simulink model "TST_InjCrv_MI1Cor"  (R2016b)
settings: Solver=FixedStepDiscrete  StartTime=0.0  StopTime=simTime  FixedStep=sampleTime  RelTol=1e-3
values from neighbouring files (symbols this model uses):
  testCase = 1    [initTST_InjCrv_MI1Cor_001.m]
libraries: simulink x3, UnitTest_Lib x1
settings Model: Creator=zhengjinyan  LastModifiedBy=zhengjinyan
settings DebuggingCC: SignalRangeChecking=error

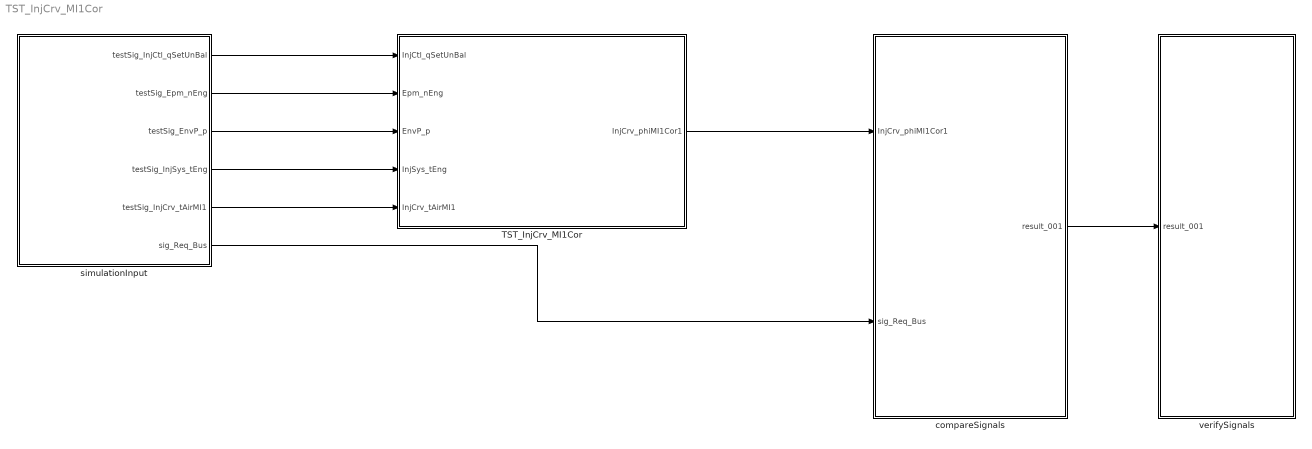
== system TST_InjCrv_MI1Cor ==
  TST_InjCrv_MI1Cor : Subsystem
  compareSignals : Subsystem
  simulationInput : Subsystem
  verifySignals : Subsystem
  wires:
  simulationInput/1(testSig_InjCtl_qSetUnBal) -> TST_InjCrv_MI1Cor/1(InjCtl_qSetUnBal)
  simulationInput/2(testSig_Epm_nEng) -> TST_InjCrv_MI1Cor/2(Epm_nEng)
  simulationInput/3(testSig_EnvP_p) -> TST_InjCrv_MI1Cor/3(EnvP_p)
  simulationInput/4(testSig_InjSys_tEng) -> TST_InjCrv_MI1Cor/4(InjSys_tEng)
  simulationInput/5(testSig_InjCrv_tAirMI1) -> TST_InjCrv_MI1Cor/5(InjCrv_tAirMI1)
  TST_InjCrv_MI1Cor/1(InjCrv_phiMI1Cor1) -> compareSignals/1(InjCrv_phiMI1Cor1)
  simulationInput/6(sig_Req_Bus) -> compareSignals/2(sig_Req_Bus)
  compareSignals/1(result_001) -> verifySignals/1(result_001)

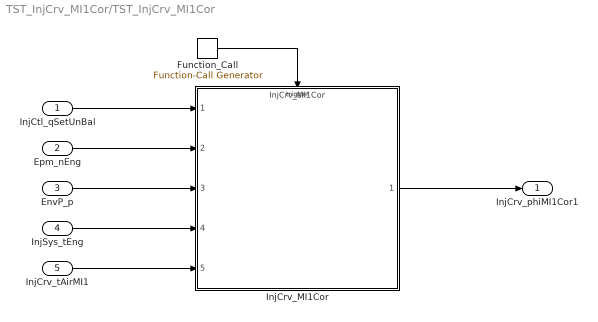
== system TST_InjCrv_MI1Cor/TST_InjCrv_MI1Cor ==
  InjCtl_qSetUnBal : Inport
  Epm_nEng : Inport  Port=2
  EnvP_p : Inport  Port=3
  InjSys_tEng : Inport  Port=4
  InjCrv_tAirMI1 : Inport  Port=5
  Function_Call : simulink/Ports & Subsystems/Function-Call Generator  sample_time=sampleTime  numberOfIterations=1
  InjCrv_MI1Cor : ModelReference  ModelNameDialog=InjCrv_MI1Cor  SimulationMode=Normal  ModelReferenceVersion=1.23  TriggerPortName=function  TriggerPortTriggerType=function-call  TriggerPortStatesWhenEnabling=held
  InjCrv_phiMI1Cor1 : Outport
  wires:
  Function_Call/1 -> InjCrv_MI1Cor/Trigger
  InjCtl_qSetUnBal/1 -> InjCrv_MI1Cor/1
  Epm_nEng/1 -> InjCrv_MI1Cor/2
  EnvP_p/1 -> InjCrv_MI1Cor/3
  InjSys_tEng/1 -> InjCrv_MI1Cor/4
  InjCrv_tAirMI1/1 -> InjCrv_MI1Cor/5
  InjCrv_MI1Cor/1 -> InjCrv_phiMI1Cor1/1

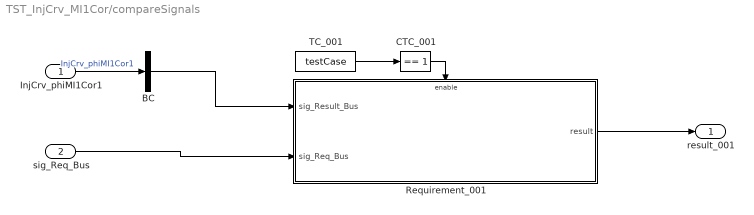
== system TST_InjCrv_MI1Cor/compareSignals ==
  InjCrv_phiMI1Cor1 : Inport
  sig_Req_Bus : Inport  Port=2
  BC : BusCreator  Inputs=1
  CTC_001 : simulink/Logic and Bit Operations/Compare To Constant  relop===  const=1  OutDataTypeStr=boolean
  Requirement_001 : Subsystem
  TC_001 : Constant  Value=testCase
  result_001 : Outport
  wires:
  InjCrv_phiMI1Cor1/1 -> BC/1  "InjCrv_phiMI1Cor1"
  TC_001/1 -> CTC_001/1
  CTC_001/1 -> Requirement_001/Enable
  sig_Req_Bus/1 -> Requirement_001/2(sig_Req_Bus)
  BC/1 -> Requirement_001/1(sig_Result_Bus)
  Requirement_001/1(result) -> result_001/1

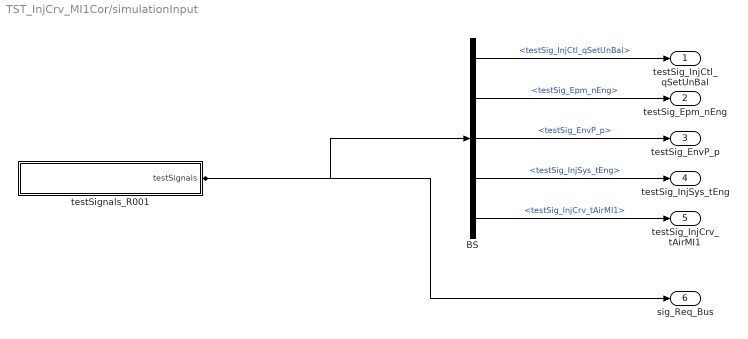
== system TST_InjCrv_MI1Cor/simulationInput ==
  BS : BusSelector  OutputSignals=testSig_InjCtl_qSetUnBal,testSig_Epm_nEng,testSig_EnvP_p,testSig_InjSys_tEng,testSig_InjCrv_tAirMI1
  testSignals_R001 : Subsystem
  testSig_InjCtl_qSetUnBal : Outport
  testSig_Epm_nEng : Outport  Port=2
  testSig_EnvP_p : Outport  Port=3
  testSig_InjSys_tEng : Outport  Port=4
  testSig_InjCrv_tAirMI1 : Outport  Port=5
  sig_Req_Bus : Outport  Port=6
  wires:
  BS/1 -> testSig_InjCtl_qSetUnBal/1  "<testSig_InjCtl_qSetUnBal>"
  BS/2 -> testSig_Epm_nEng/1  "<testSig_Epm_nEng>"
  BS/3 -> testSig_EnvP_p/1  "<testSig_EnvP_p>"
  BS/4 -> testSig_InjSys_tEng/1  "<testSig_InjSys_tEng>"
  BS/5 -> testSig_InjCrv_tAirMI1/1  "<testSig_InjCrv_tAirMI1>"
  testSignals_R001/1(testSignals) -> BS/1, sig_Req_Bus/1

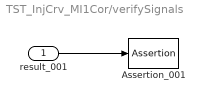
== system TST_InjCrv_MI1Cor/verifySignals ==
  result_001 : Inport
  Assertion_001 : Assertion  Enabled=off
  wires:
  result_001/1 -> Assertion_001/1

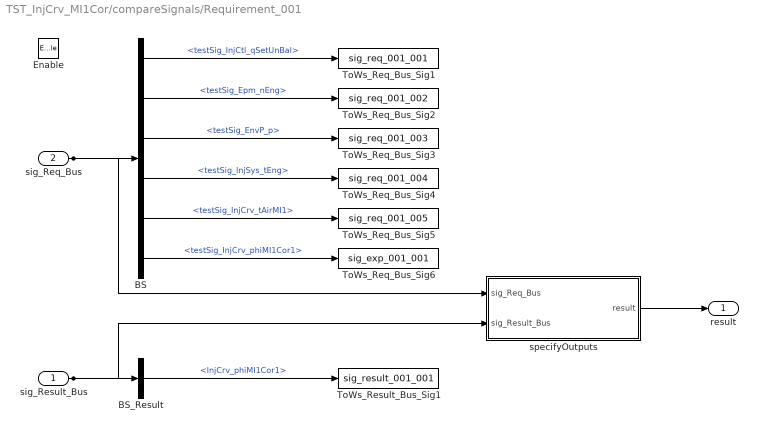
== system TST_InjCrv_MI1Cor/compareSignals/Requirement_001 ==
  sig_Result_Bus : Inport
  sig_Req_Bus : Inport  Port=2
  Enable : EnablePort
  BS : BusSelector  OutputSignals=testSig_InjCtl_qSetUnBal,testSig_Epm_nEng,testSig_EnvP_p,testSig_InjSys_tEng,testSig_InjCrv_tAirMI1,testSig_InjCrv_phiMI1Cor1
  BS_Result : BusSelector  OutputSignals=InjCrv_phiMI1Cor1
  ToWs_Req_Bus_Sig1 : ToWorkspace  VariableName=sig_req_001_001  SaveFormat=Structure With Time
  ToWs_Req_Bus_Sig2 : ToWorkspace  VariableName=sig_req_001_002  SaveFormat=Structure With Time
  ToWs_Req_Bus_Sig3 : ToWorkspace  VariableName=sig_req_001_003  SaveFormat=Structure With Time
  ToWs_Req_Bus_Sig4 : ToWorkspace  VariableName=sig_req_001_004  SaveFormat=Structure With Time
  ToWs_Req_Bus_Sig5 : ToWorkspace  VariableName=sig_req_001_005  SaveFormat=Structure With Time
  ToWs_Req_Bus_Sig6 : ToWorkspace  VariableName=sig_exp_001_001  SaveFormat=Structure With Time
  ToWs_Result_Bus_Sig1 : ToWorkspace  VariableName=sig_result_001_001  SaveFormat=Structure With Time
  specifyOutputs : Subsystem
  result : Outport
  wires:
  sig_Req_Bus/1 -> BS/1, specifyOutputs/1(sig_Req_Bus)
  BS/1 -> ToWs_Req_Bus_Sig1/1  "<testSig_InjCtl_qSetUnBal>"
  BS/2 -> ToWs_Req_Bus_Sig2/1  "<testSig_Epm_nEng>"
  BS/3 -> ToWs_Req_Bus_Sig3/1  "<testSig_EnvP_p>"
  BS/4 -> ToWs_Req_Bus_Sig4/1  "<testSig_InjSys_tEng>"
  BS/5 -> ToWs_Req_Bus_Sig5/1  "<testSig_InjCrv_tAirMI1>"
  BS/6 -> ToWs_Req_Bus_Sig6/1  "<testSig_InjCrv_phiMI1Cor1>"
  sig_Result_Bus/1 -> BS_Result/1, specifyOutputs/2(sig_Result_Bus)
  BS_Result/1 -> ToWs_Result_Bus_Sig1/1  "<InjCrv_phiMI1Cor1>"
  specifyOutputs/1(result) -> result/1

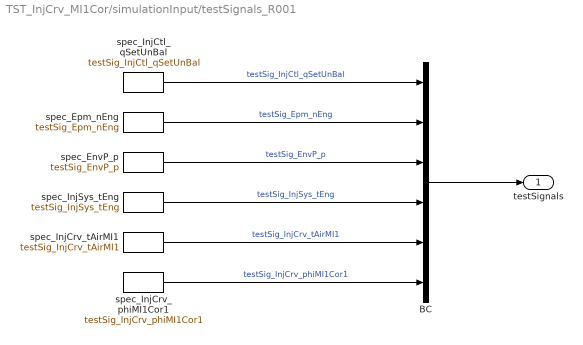
== system TST_InjCrv_MI1Cor/simulationInput/testSignals_R001 ==
  BC : BusCreator  Inputs=6
  spec_EnvP_p : FromWorkspace  VariableName=testSig_EnvP_p  Interpolate=off  OutputAfterFinalValue=Holding final value
  spec_Epm_nEng : FromWorkspace  VariableName=testSig_Epm_nEng  Interpolate=off  OutputAfterFinalValue=Holding final value
  spec_InjCrv_phiMI1Cor1 : FromWorkspace  VariableName=testSig_InjCrv_phiMI1Cor1  Interpolate=off  OutputAfterFinalValue=Holding final value
  spec_InjCrv_tAirMI1 : FromWorkspace  VariableName=testSig_InjCrv_tAirMI1  Interpolate=off  OutputAfterFinalValue=Holding final value
  spec_InjCtl_qSetUnBal : FromWorkspace  VariableName=testSig_InjCtl_qSetUnBal  Interpolate=off  OutputAfterFinalValue=Holding final value
  spec_InjSys_tEng : FromWorkspace  VariableName=testSig_InjSys_tEng  Interpolate=off  OutputAfterFinalValue=Holding final value
  testSignals : Outport
  wires:
  BC/1 -> testSignals/1
  spec_InjCtl_qSetUnBal/1 -> BC/1  "testSig_InjCtl_qSetUnBal"
  spec_Epm_nEng/1 -> BC/2  "testSig_Epm_nEng"
  spec_EnvP_p/1 -> BC/3  "testSig_EnvP_p"
  spec_InjSys_tEng/1 -> BC/4  "testSig_InjSys_tEng"
  spec_InjCrv_tAirMI1/1 -> BC/5  "testSig_InjCrv_tAirMI1"
  spec_InjCrv_phiMI1Cor1/1 -> BC/6  "testSig_InjCrv_phiMI1Cor1"

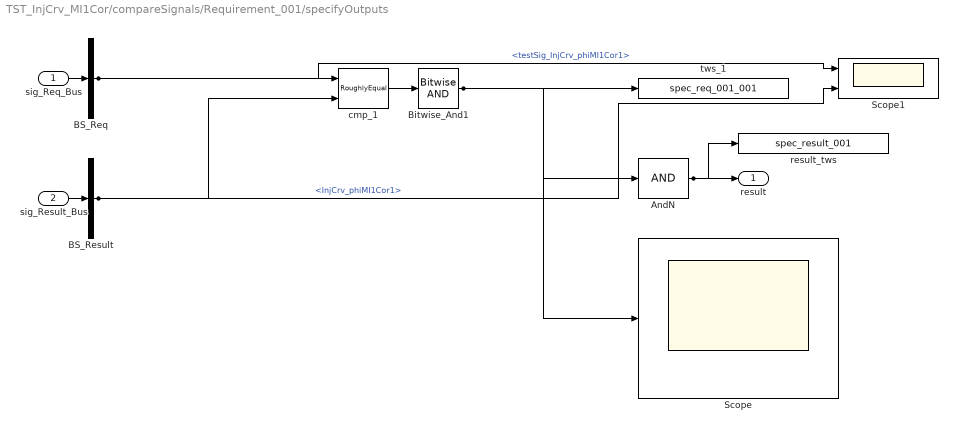
== system TST_InjCrv_MI1Cor/compareSignals/Requirement_001/specifyOutputs ==
  sig_Req_Bus : Inport
  sig_Result_Bus : Inport  Port=2
  AndN : Logic  Inputs=1
  BS_Req : BusSelector  OutputSignals=testSig_InjCrv_phiMI1Cor1
  BS_Result : BusSelector  OutputSignals=InjCrv_phiMI1Cor1
  Bitwise_And1 : simulink/Logic and Bit Operations/Bitwise Operator  logicop=AND  UseBitMask=off  BitMask=bin2dec('11011001')  BitMaskRealWorld=Stored Integer
  Scope : Scope
  Scope1 : Scope  NumInputPorts=2
  cmp_1 : UnitTest_Lib/RoughlyEqual  slope=0.1
  result_tws : ToWorkspace  VariableName=spec_result_001
  tws_1 : ToWorkspace  VariableName=spec_req_001_001
  result : Outport
  wires:
  sig_Req_Bus/1 -> BS_Req/1
  sig_Result_Bus/1 -> BS_Result/1
  AndN/1 -> result/1, result_tws/1
  BS_Req/1 -> cmp_1/1, Scope1/1  "<testSig_InjCrv_phiMI1Cor1>"
  BS_Result/1 -> cmp_1/2, Scope1/2  "<InjCrv_phiMI1Cor1>"
  cmp_1/1 -> Bitwise_And1/1
  Bitwise_And1/1 -> tws_1/1, AndN/1, Scope/1
